simulink model "harmonic_analysis"  (R2016a)
settings: Solver=VariableStepAuto  StartTime=0.0  StopTime=Tfinal  RelTol=1e-3
values from neighbouring files (symbols this model uses):
  Ts = 0.1e-6    (= 1e-07)    [cizdir.m]
libraries: powerlib_meascontrol x80, powerlib x1
settings Model: SimulationMode=accelerator  Creator=mesutto  LastModifiedBy=mesutto

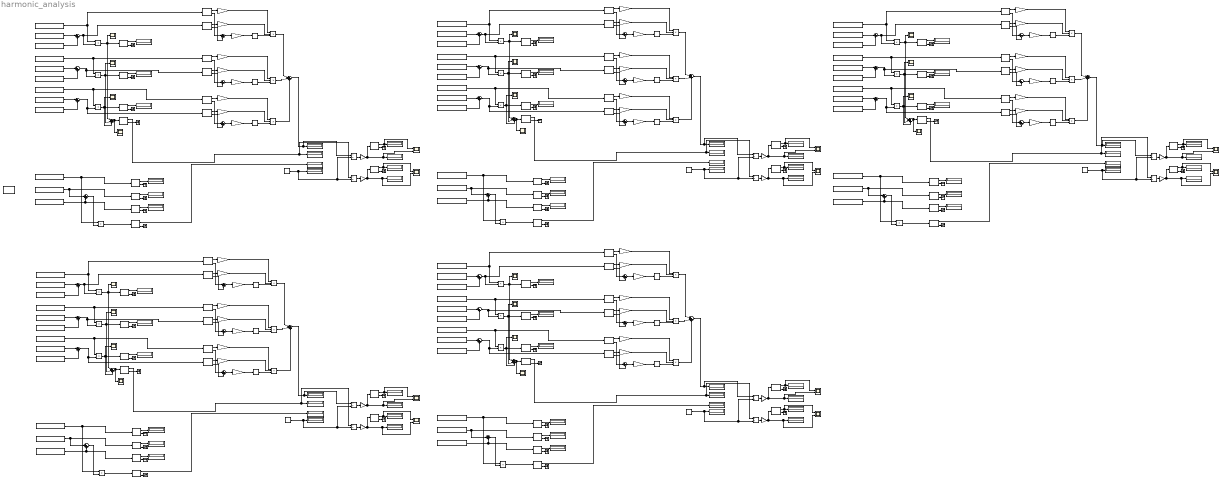
== system harmonic_analysis ==
  Constant : Constant  Value=398
  Constant1 : Constant  Value=775
  Constant2 : Constant  Value=1150
  Constant3 : Constant  Value=1530
  Constant4 : Constant  Value=1910
  Display{1..64,66..71} (70 alike) : Display
  Divide{1..4,8..9,12..13,17,19} (10 alike) : Product  Inputs=*/
  Fourier{1..6,8..12,24..29,31,36..41,43,45,50..55,57,59,64..69,71..80} (50 alike) : powerlib_meascontrol/Measurements/Fourier  Freq=freq_fourier  n=0  InInit=[0, 0]  Ts=0
  Fourier{7,13..23,30,32..35,42,44,46..49,56,58,60..63,70} (30 alike) : powerlib_meascontrol/Measurements/Fourier  Freq=50  n=1  InInit=[0, 0]  Ts=0
  From Workspace1 : FromWorkspace  VariableName=[time_DCload5*1e-3 Va_load1]  OutDataTypeStr=double  SampleTime=Ts
  From Workspace10 : FromWorkspace  VariableName=[time_DC_a1_load5*1e-3 Idc_a1_load1]  OutDataTypeStr=double  SampleTime=Ts
  From Workspace11 : FromWorkspace  VariableName=[time_DC_a2_load5*1e-3 Idc_a2_load1]  OutDataTypeStr=double  SampleTime=Ts
  From Workspace12 : FromWorkspace  VariableName=[time_DCload5*1e-3 Va_load2]  OutDataTypeStr=double  SampleTime=Ts
  From Workspace13 : FromWorkspace  VariableName=[time_DCload5*1e-3 Ic_a2_load1]  OutDataTypeStr=double  SampleTime=Ts
  From Workspace14 : FromWorkspace  VariableName=[time_DC_a1_load5*1e-3 Idc_a1_load2]  OutDataTypeStr=double  SampleTime=Ts
  From Workspace15 : FromWorkspace  VariableName=[time_DC_a2_load5*1e-3 Idc_a2_load2]  OutDataTypeStr=double  SampleTime=Ts
  From Workspace16 : FromWorkspace  VariableName=[time_DCload5*1e-3 Ic_a2_load2]  OutDataTypeStr=double  SampleTime=Ts
  From Workspace17 : FromWorkspace  VariableName=[time_DCload5*1e-3 Ia_a1_load2]  OutDataTypeStr=double  SampleTime=Ts
  From Workspace18 : FromWorkspace  VariableName=[time_DCload5*1e-3 Ia_a2_load2]  OutDataTypeStr=double  SampleTime=Ts
  From Workspace19 : FromWorkspace  VariableName=[time_DCload5*1e-3 Vb_load2]  OutDataTypeStr=double  SampleTime=Ts
  From Workspace2 : FromWorkspace  VariableName=[time_DCload5*1e-3 Ia_a1_load1]  OutDataTypeStr=double  SampleTime=Ts
  From Workspace20 : FromWorkspace  VariableName=[time_DCload5*1e-3 Ib_a1_load2]  OutDataTypeStr=double  SampleTime=Ts
  From Workspace21 : FromWorkspace  VariableName=[time_DCload5*1e-3 Ib_a2_load2]  OutDataTypeStr=double  SampleTime=Ts
  From Workspace22 : FromWorkspace  VariableName=[time_DCload5*1e-3 Vc_load2]  OutDataTypeStr=double  SampleTime=Ts
  From Workspace23 : FromWorkspace  VariableName=[time_DCload5*1e-3 Ic_a1_load2]  OutDataTypeStr=double  SampleTime=Ts
  From Workspace24 : FromWorkspace  VariableName=[time_DCload5*1e-3 Vdc_load2]  OutDataTypeStr=double  SampleTime=Ts
  From Workspace25 : FromWorkspace  VariableName=[time_DCload5*1e-3 Va_load3]  OutDataTypeStr=double  SampleTime=Ts
  From Workspace26 : FromWorkspace  VariableName=[time_DC_a1_load5*1e-3 Idc_a1_load3]  OutDataTypeStr=double  SampleTime=Ts
  From Workspace27 : FromWorkspace  VariableName=[time_DC_a2_load5*1e-3 Idc_a2_load3]  OutDataTypeStr=double  SampleTime=Ts
  From Workspace28 : FromWorkspace  VariableName=[time_DCload5*1e-3 Ic_a2_load3]  OutDataTypeStr=double  SampleTime=Ts
  From Workspace29 : FromWorkspace  VariableName=[time_DCload5*1e-3 Ia_a1_load3]  OutDataTypeStr=double  SampleTime=Ts
  From Workspace3 : FromWorkspace  VariableName=[time_DCload5*1e-3 Ia_a2_load1]  OutDataTypeStr=double  SampleTime=Ts
  From Workspace30 : FromWorkspace  VariableName=[time_DCload5*1e-3 Ia_a2_load3]  OutDataTypeStr=double  SampleTime=Ts
  From Workspace31 : FromWorkspace  VariableName=[time_DCload5*1e-3 Vb_load3]  OutDataTypeStr=double  SampleTime=Ts
  From Workspace32 : FromWorkspace  VariableName=[time_DCload5*1e-3 Ib_a1_load3]  OutDataTypeStr=double  SampleTime=Ts
  From Workspace33 : FromWorkspace  VariableName=[time_DCload5*1e-3 Ib_a2_load3]  OutDataTypeStr=double  SampleTime=Ts
  From Workspace34 : FromWorkspace  VariableName=[time_DCload5*1e-3 Vc_load3]  OutDataTypeStr=double  SampleTime=Ts
  From Workspace35 : FromWorkspace  VariableName=[time_DCload5*1e-3 Ic_a1_load3]  OutDataTypeStr=double  SampleTime=Ts
  From Workspace36 : FromWorkspace  VariableName=[time_DCload5*1e-3 Vdc_load3]  OutDataTypeStr=double  SampleTime=Ts
  From Workspace37 : FromWorkspace  VariableName=[time_DCload5*1e-3 Va_load4]  OutDataTypeStr=double  SampleTime=Ts
  From Workspace38 : FromWorkspace  VariableName=[time_DC_a1_load5*1e-3 Idc_a1_load4]  OutDataTypeStr=double  SampleTime=Ts
  From Workspace39 : FromWorkspace  VariableName=[time_DC_a2_load5*1e-3 Idc_a2_load4]  OutDataTypeStr=double  SampleTime=Ts
  From Workspace4 : FromWorkspace  VariableName=[time_DCload5*1e-3 Vb_load1]  OutDataTypeStr=double  SampleTime=Ts
  From Workspace40 : FromWorkspace  VariableName=[time_DCload5*1e-3 Ic_a2_load4]  OutDataTypeStr=double  SampleTime=Ts
  From Workspace41 : FromWorkspace  VariableName=[time_DCload5*1e-3 Ia_a1_load4]  OutDataTypeStr=double  SampleTime=Ts
  From Workspace42 : FromWorkspace  VariableName=[time_DCload5*1e-3 Ia_a2_load4]  OutDataTypeStr=double  SampleTime=Ts
  From Workspace43 : FromWorkspace  VariableName=[time_DCload5*1e-3 Vb_load4]  OutDataTypeStr=double  SampleTime=Ts
  From Workspace44 : FromWorkspace  VariableName=[time_DCload5*1e-3 Ib_a1_load4]  OutDataTypeStr=double  SampleTime=Ts
  From Workspace45 : FromWorkspace  VariableName=[time_DCload5*1e-3 Ib_a2_load4]  OutDataTypeStr=double  SampleTime=Ts
  From Workspace46 : FromWorkspace  VariableName=[time_DCload5*1e-3 Vc_load4]  OutDataTypeStr=double  SampleTime=Ts
  From Workspace47 : FromWorkspace  VariableName=[time_DCload5*1e-3 Ic_a1_load4]  OutDataTypeStr=double  SampleTime=Ts
  From Workspace48 : FromWorkspace  VariableName=[time_DCload5*1e-3 Vdc_load4]  OutDataTypeStr=double  SampleTime=Ts
  From Workspace49 : FromWorkspace  VariableName=[time_DCload5*1e-3 Va_load5]  OutDataTypeStr=double  SampleTime=Ts
  From Workspace5 : FromWorkspace  VariableName=[time_DCload5*1e-3 Ib_a1_load1]  OutDataTypeStr=double  SampleTime=Ts
  From Workspace50 : FromWorkspace  VariableName=[time_DC_a1_load5*1e-3 Idc_a1_load5]  OutDataTypeStr=double  SampleTime=Ts
  From Workspace51 : FromWorkspace  VariableName=[time_DC_a2_load5*1e-3 Idc_a2_load5]  OutDataTypeStr=double  SampleTime=Ts
  From Workspace52 : FromWorkspace  VariableName=[time_DCload5*1e-3 Ic_a2_load5]  OutDataTypeStr=double  SampleTime=Ts
  From Workspace53 : FromWorkspace  VariableName=[time_DCload5*1e-3 Ia_a1_load5]  OutDataTypeStr=double  SampleTime=Ts
  From Workspace54 : FromWorkspace  VariableName=[time_DCload5*1e-3 Ia_a2_load5]  OutDataTypeStr=double  SampleTime=Ts
  From Workspace55 : FromWorkspace  VariableName=[time_DCload5*1e-3 Vb_load5]  OutDataTypeStr=double  SampleTime=Ts
  From Workspace56 : FromWorkspace  VariableName=[time_DCload5*1e-3 Ib_a1_load5]  OutDataTypeStr=double  SampleTime=Ts
  From Workspace57 : FromWorkspace  VariableName=[time_DCload5*1e-3 Ib_a2_load5]  OutDataTypeStr=double  SampleTime=Ts
  From Workspace58 : FromWorkspace  VariableName=[time_DCload5*1e-3 Vc_load5]  OutDataTypeStr=double  SampleTime=Ts
  From Workspace59 : FromWorkspace  VariableName=[time_DCload5*1e-3 Ic_a1_load5]  OutDataTypeStr=double  SampleTime=Ts
  From Workspace6 : FromWorkspace  VariableName=[time_DCload5*1e-3 Ib_a2_load1]  OutDataTypeStr=double  SampleTime=Ts
  From Workspace60 : FromWorkspace  VariableName=[time_DCload5*1e-3 Vdc_load5]  OutDataTypeStr=double  SampleTime=Ts
  From Workspace7 : FromWorkspace  VariableName=[time_DCload5*1e-3 Vc_load1]  OutDataTypeStr=double  SampleTime=Ts
  From Workspace8 : FromWorkspace  VariableName=[time_DCload5*1e-3 Ic_a1_load1]  OutDataTypeStr=double  SampleTime=Ts
  From Workspace9 : FromWorkspace  VariableName=[time_DCload5*1e-3 Vdc_load1]  OutDataTypeStr=double  SampleTime=Ts
  Gain{1..4,32..33,45..46,58,63} (10 alike) : Gain  Gain=100
  Gain{5..6,10..11,14,19,29,38..39,42,51..52,55,64..65} (15 alike) : Gain  Gain=pi/180
  Gain{8..9,12..13,15..18,20..21,25..28,30..31,35..36,40..41,43..44,48..49,53..54,56..57,61..62} (30 alike) : Gain  Gain=1/sqrt(2)
  Product{1..5,9..11,15..17,21..24,28..31,35} (20 alike) : Product
  Product{6..8,12..14,18..20,25..27,32..34} (15 alike) : Product  Inputs=3
  Scope{1..4,9..12,17..19,24..27,32..35,40} (20 alike) : Scope
  Scope{5..8,20..21,28..29,36..37} (10 alike) : Scope  NumInputPorts=2
  Sum{1,8..10,17..19,25..26,28,34..35,37,43..44} (15 alike) : Sum  Inputs=|+-
  Sum{2,7,11,16,24,27,33,36,42,45} (10 alike) : Sum  Inputs=|+++
  Sum{3..6,12..15,20..23,29..32,38..41} (20 alike) : Sum  Inputs=|++
  Terminator{,1..49} (50 alike) : Terminator
  Trigonometric Function{1..15} (15 alike) : Trigonometry  Operator=cos
  powergui : powerlib/powergui  Priority=1  SimulationMode=Discrete  SolverType=Tustin/Backward Euler (TBE)  SampleTime=Ts  frequency=60  SPID=off  DisableSnubberDevices=off  DisableRonSwitches=off  DisableVfSwitches=off  SwTol=0  DisplayEquations=off  Interpol=off  ExternalGateDelay=off  methode=off  Ts=10  FunctionMessages=off  echomessages=off  HookPort=off  EnableUseOfTLC=off  x0status=blocks  frequencyindice=60  Pbase=100e6  ErrMax=1e-4  Iterations=50  UnitsV=kV  UnitsW=MW  buscounter=0  RestoreLinks=warning  ResistiveCurrentMeasurement=off  Frange=[0:2:500]  Ylog=off  Xlog=on  ShowGrid=off  save=off  variable=ZData  structure=Pa  ZoomFFT=off  StartTime=0.005  cycles=3  DisplayStyle=5  fundamental=100  FreqAxis=off  MaxFrequency=200000  frequencyindicesteady=1  RmsSteady=1  display=off
  wires:
  Fourier4/1 -> Display11/1
  Fourier4/2 -> Terminator/1
  From Workspace10/1 -> Sum3/1, Fourier5/1
  Fourier5/1 -> Display12/1
  Fourier5/2 -> Terminator1/1
  From Workspace11/1 -> Sum3/2, Fourier6/1
  Fourier6/1 -> Display13/1
  Fourier6/2 -> Terminator2/1
  Fourier8/2 -> Terminator4/1
  Sum3/1 -> Product2/2
  Product2/1 -> Fourier8/1
  From Workspace9/1 -> Product2/1, Fourier4/1
  From Workspace2/1 -> Sum4/1
  From Workspace3/1 -> Sum4/2
  From Workspace1/1 -> Fourier13/1, Product3/1
  From Workspace5/1 -> Sum5/1
  From Workspace6/1 -> Sum5/2
  Sum5/1 -> Product4/2, Fourier16/1
  From Workspace4/1 -> Fourier15/1, Product4/1
  From Workspace8/1 -> Sum6/1
  From Workspace13/1 -> Sum6/2
  Sum6/1 -> Fourier18/1, Product5/2
  Fourier9/1 -> Display16/1
  Fourier9/2 -> Terminator5/1
  Fourier10/1 -> Display17/1
  Fourier10/2 -> Terminator6/1
  Fourier11/1 -> Display18/1
  Fourier11/2 -> Terminator7/1
  Product3/1 -> Scope1/1, Sum7/1, Fourier9/1
  Product4/1 -> Scope2/1, Sum7/2, Fourier10/1
  Product5/1 -> Scope3/1, Sum7/3, Fourier11/1
  Fourier12/2 -> Terminator8/1
  Sum7/1 -> Scope4/1, Fourier12/1
  Fourier13/1 -> Gain8/1
  Fourier14/1 -> Gain9/1
  Sum4/1 -> Fourier14/1, Product3/2
  Fourier13/2 -> Sum8/1
  Fourier14/2 -> Sum8/2
  Sum8/1 -> Gain10/1
  Gain10/1 -> Trigonometric Function2/1
  Trigonometric Function2/1 -> Product6/3
  Gain9/1 -> Product6/2
  Gain8/1 -> Product6/1
  Fourier15/1 -> Gain12/1
  Fourier16/1 -> Gain13/1
  Fourier15/2 -> Sum9/1
  Fourier16/2 -> Sum9/2
  Sum9/1 -> Gain11/1
  Gain11/1 -> Trigonometric Function3/1
  Trigonometric Function3/1 -> Product7/3
  Gain13/1 -> Product7/2
  Gain12/1 -> Product7/1
  Fourier17/1 -> Gain15/1
  Fourier18/1 -> Gain16/1
  Fourier17/2 -> Sum10/1
  Fourier18/2 -> Sum10/2
  Sum10/1 -> Gain14/1
  Gain14/1 -> Trigonometric Function4/1
  Trigonometric Function4/1 -> Product8/3
  Gain16/1 -> Product8/2
  Gain15/1 -> Product8/1
  From Workspace7/1 -> Fourier17/1, Product5/1
  Product6/1 -> Sum11/1
  Product7/1 -> Sum11/2
  Product8/1 -> Sum11/3
  Fourier8/1 -> Display15/1
  Fourier24/1 -> Display7/1
  Fourier24/2 -> Terminator3/1
  From Workspace14/1 -> Sum12/1, Fourier25/1
  Fourier25/1 -> Display8/1
  Fourier25/2 -> Terminator9/1
  From Workspace15/1 -> Sum12/2, Fourier26/1
  Fourier26/1 -> Display9/1
  Fourier26/2 -> Terminator10/1
  Fourier27/2 -> Terminator11/1
  Sum12/1 -> Product1/2
  Product1/1 -> Fourier27/1
  From Workspace24/1 -> Product1/1, Fourier24/1
  From Workspace17/1 -> Sum13/1
  From Workspace18/1 -> Sum13/2
  From Workspace12/1 -> Fourier7/1, Product9/1
  From Workspace20/1 -> Sum14/1
  From Workspace21/1 -> Sum14/2
  Sum14/1 -> Product10/2, Fourier21/1
  From Workspace19/1 -> Fourier20/1, Product10/1
  From Workspace23/1 -> Sum15/1
  From Workspace16/1 -> Sum15/2
  Sum15/1 -> Fourier23/1, Product11/2
  Fourier28/1 -> Display14/1
  Fourier28/2 -> Terminator12/1
  Fourier1/1 -> Display20/1
  Fourier1/2 -> Terminator13/1
  Fourier2/1 -> Display22/1
  Fourier2/2 -> Terminator14/1
  Product9/1 -> Scope9/1, Sum16/1, Fourier28/1
  Product10/1 -> Scope10/1, Sum16/2, Fourier1/1
  Product11/1 -> Scope11/1, Sum16/3, Fourier2/1
  Fourier3/2 -> Terminator15/1
  Sum16/1 -> Scope12/1, Fourier3/1
  Fourier7/1 -> Gain25/1
  Fourier19/1 -> Gain26/1
  Sum13/1 -> Fourier19/1, Product9/2
  Fourier7/2 -> Sum17/1
  Fourier19/2 -> Sum17/2
  Sum17/1 -> Gain5/1
  Gain5/1 -> Trigonometric Function1/1
  Trigonometric Function1/1 -> Product12/3
  Gain26/1 -> Product12/2
  Gain25/1 -> Product12/1
  Fourier20/1 -> Gain17/1
  Fourier21/1 -> Gain18/1
  Fourier20/2 -> Sum18/1
  Fourier21/2 -> Sum18/2
  Sum18/1 -> Gain6/1
  Gain6/1 -> Trigonometric Function5/1
  Trigonometric Function5/1 -> Product13/3
  Gain18/1 -> Product13/2
  Gain17/1 -> Product13/1
  Fourier22/1 -> Gain20/1
  Fourier23/1 -> Gain21/1
  Fourier22/2 -> Sum1/1
  Fourier23/2 -> Sum1/2
  Sum1/1 -> Gain19/1
  Gain19/1 -> Trigonometric Function6/1
  Trigonometric Function6/1 -> Product14/3
  Gain21/1 -> Product14/2
  Gain20/1 -> Product14/1
  From Workspace22/1 -> Fourier22/1, Product11/1
  Product12/1 -> Sum2/1
  Product13/1 -> Sum2/2
  Product14/1 -> Sum2/3
  Fourier27/1 -> Display10/1
  Fourier36/1 -> Display40/1
  Fourier36/2 -> Terminator22/1
  From Workspace26/1 -> Sum20/1, Fourier37/1
  Fourier37/1 -> Display41/1
  Fourier37/2 -> Terminator23/1
  From Workspace27/1 -> Sum20/2, Fourier38/1
  Fourier38/1 -> Display42/1
  Fourier38/2 -> Terminator16/1
  Fourier39/2 -> Terminator17/1
  Sum20/1 -> Product15/2
  Product15/1 -> Fourier39/1
  From Workspace36/1 -> Product15/1, Fourier36/1
  From Workspace29/1 -> Sum21/1
  From Workspace30/1 -> Sum21/2
  From Workspace25/1 -> Fourier42/1, Product21/1
  From Workspace32/1 -> Sum22/1
  From Workspace33/1 -> Sum22/2
  Sum22/1 -> Product16/2, Fourier33/1
  From Workspace31/1 -> Fourier32/1, Product16/1
  From Workspace35/1 -> Sum23/1
  From Workspace28/1 -> Sum23/2
  Sum23/1 -> Fourier35/1, Product17/2
  Fourier40/1 -> Display30/1
  Fourier40/2 -> Terminator18/1
  Fourier29/1 -> Display31/1
  Fourier29/2 -> Terminator19/1
  Fourier31/1 -> Display32/1
  Fourier31/2 -> Terminator20/1
  Product21/1 -> Scope24/1, Sum24/1, Fourier40/1
  Product16/1 -> Scope17/1, Sum24/2, Fourier29/1
  Product17/1 -> Scope18/1, Sum24/3, Fourier31/1
  Fourier41/2 -> Terminator21/1
  Sum24/1 -> Scope19/1, Fourier41/1
  Fourier42/1 -> Gain35/1
  Fourier30/1 -> Gain36/1
  Sum21/1 -> Fourier30/1, Product21/2
  Fourier42/2 -> Sum25/1
  Fourier30/2 -> Sum25/2
  Sum25/1 -> Gain38/1
  Gain38/1 -> Trigonometric Function7/1
  Trigonometric Function7/1 -> Product18/3
  Gain36/1 -> Product18/2
  Gain35/1 -> Product18/1
  Fourier32/1 -> Gain27/1
  Fourier33/1 -> Gain28/1
  Fourier32/2 -> Sum26/1
  Fourier33/2 -> Sum26/2
  Sum26/1 -> Gain39/1
  Gain39/1 -> Trigonometric Function8/1
  Trigonometric Function8/1 -> Product19/3
  Gain28/1 -> Product19/2
  Gain27/1 -> Product19/1
  Fourier34/1 -> Gain30/1
  Fourier35/1 -> Gain31/1
  Fourier34/2 -> Sum19/1
  Fourier35/2 -> Sum19/2
  Sum19/1 -> Gain29/1
  Gain29/1 -> Trigonometric Function9/1
  Trigonometric Function9/1 -> Product20/3
  Gain31/1 -> Product20/2
  Gain30/1 -> Product20/1
  From Workspace34/1 -> Fourier34/1, Product17/1
  Product18/1 -> Sum27/1
  Product19/1 -> Sum27/2
  Product20/1 -> Sum27/3
  Fourier39/1 -> Display29/1
  Fourier50/1 -> Display54/1
  Fourier50/2 -> Terminator30/1
  From Workspace38/1 -> Sum29/1, Fourier51/1
  Fourier51/1 -> Display55/1
  Fourier51/2 -> Terminator31/1
  From Workspace39/1 -> Sum29/2, Fourier52/1
  Fourier52/1 -> Display56/1
  Fourier52/2 -> Terminator24/1
  Fourier53/2 -> Terminator25/1
  Sum29/1 -> Product22/2
  Product22/1 -> Fourier53/1
  From Workspace48/1 -> Product22/1, Fourier50/1
  From Workspace41/1 -> Sum30/1
  From Workspace42/1 -> Sum30/2
  From Workspace37/1 -> Fourier56/1, Product28/1
  From Workspace44/1 -> Sum31/1
  From Workspace45/1 -> Sum31/2
  Sum31/1 -> Product23/2, Fourier47/1
  From Workspace43/1 -> Fourier46/1, Product23/1
  From Workspace47/1 -> Sum32/1
  From Workspace40/1 -> Sum32/2
  Sum32/1 -> Fourier49/1, Product24/2
  Fourier54/1 -> Display44/1
  Fourier54/2 -> Terminator26/1
  Fourier43/1 -> Display45/1
  Fourier43/2 -> Terminator27/1
  Fourier45/1 -> Display46/1
  Fourier45/2 -> Terminator28/1
  Product28/1 -> Scope32/1, Sum33/1, Fourier54/1
  Product23/1 -> Scope25/1, Sum33/2, Fourier43/1
  Product24/1 -> Scope26/1, Sum33/3, Fourier45/1
  Fourier55/2 -> Terminator29/1
  Sum33/1 -> Scope27/1, Fourier55/1
  Fourier56/1 -> Gain48/1
  Fourier44/1 -> Gain49/1
  Sum30/1 -> Fourier44/1, Product28/2
  Fourier56/2 -> Sum34/1
  Fourier44/2 -> Sum34/2
  Sum34/1 -> Gain51/1
  Gain51/1 -> Trigonometric Function10/1
  Trigonometric Function10/1 -> Product25/3
  Gain49/1 -> Product25/2
  Gain48/1 -> Product25/1
  Fourier46/1 -> Gain40/1
  Fourier47/1 -> Gain41/1
  Fourier46/2 -> Sum35/1
  Fourier47/2 -> Sum35/2
  Sum35/1 -> Gain52/1
  Gain52/1 -> Trigonometric Function11/1
  Trigonometric Function11/1 -> Product26/3
  Gain41/1 -> Product26/2
  Gain40/1 -> Product26/1
  Fourier48/1 -> Gain43/1
  Fourier49/1 -> Gain44/1
  Fourier48/2 -> Sum28/1
  Fourier49/2 -> Sum28/2
  Sum28/1 -> Gain42/1
  Gain42/1 -> Trigonometric Function12/1
  Trigonometric Function12/1 -> Product27/3
  Gain44/1 -> Product27/2
  Gain43/1 -> Product27/1
  From Workspace46/1 -> Fourier48/1, Product24/1
  Product25/1 -> Sum36/1
  Product26/1 -> Sum36/2
  Product27/1 -> Sum36/3
  Fourier53/1 -> Display43/1
  Fourier64/1 -> Display68/1
  Fourier64/2 -> Terminator38/1
  From Workspace50/1 -> Sum38/1, Fourier65/1
  Fourier65/1 -> Display69/1
  Fourier65/2 -> Terminator39/1
  From Workspace51/1 -> Sum38/2, Fourier66/1
  Fourier66/1 -> Display70/1
  Fourier66/2 -> Terminator32/1
  Fourier67/2 -> Terminator33/1
  Sum38/1 -> Product29/2
  Product29/1 -> Fourier67/1
  From Workspace60/1 -> Product29/1, Fourier64/1
  From Workspace53/1 -> Sum39/1
  From Workspace54/1 -> Sum39/2
  From Workspace49/1 -> Fourier70/1, Product35/1
  From Workspace56/1 -> Sum40/1
  From Workspace57/1 -> Sum40/2
  Sum40/1 -> Product30/2, Fourier61/1
  From Workspace55/1 -> Fourier60/1, Product30/1
  From Workspace59/1 -> Sum41/1
  From Workspace52/1 -> Sum41/2
  Sum41/1 -> Fourier63/1, Product31/2
  Fourier68/1 -> Display58/1
  Fourier68/2 -> Terminator34/1
  Fourier57/1 -> Display59/1
  Fourier57/2 -> Terminator35/1
  Fourier59/1 -> Display60/1
  Fourier59/2 -> Terminator36/1
  Product35/1 -> Scope40/1, Sum42/1, Fourier68/1
  Product30/1 -> Scope33/1, Sum42/2, Fourier57/1
  Product31/1 -> Scope34/1, Sum42/3, Fourier59/1
  Fourier69/1 -> Divide17/1, Display61/1
  Fourier69/2 -> Terminator37/1
  Sum42/1 -> Scope35/1, Fourier69/1
  Fourier70/1 -> Gain61/1
  Fourier58/1 -> Gain62/1
  Sum39/1 -> Fourier58/1, Product35/2
  Fourier70/2 -> Sum43/1
  Fourier58/2 -> Sum43/2
  Sum43/1 -> Gain64/1
  Gain64/1 -> Trigonometric Function13/1
  Trigonometric Function13/1 -> Product32/3
  Gain62/1 -> Product32/2
  Gain61/1 -> Product32/1
  Fourier60/1 -> Gain53/1
  Fourier61/1 -> Gain54/1
  Fourier60/2 -> Sum44/1
  Fourier61/2 -> Sum44/2
  Sum44/1 -> Gain65/1
  Gain65/1 -> Trigonometric Function14/1
  Trigonometric Function14/1 -> Product33/3
  Gain54/1 -> Product33/2
  Gain53/1 -> Product33/1
  Fourier62/1 -> Gain56/1
  Fourier63/1 -> Gain57/1
  Fourier62/2 -> Sum37/1
  Fourier63/2 -> Sum37/2
  Sum37/1 -> Gain55/1
  Gain55/1 -> Trigonometric Function15/1
  Trigonometric Function15/1 -> Product34/3
  Gain57/1 -> Product34/2
  Gain56/1 -> Product34/1
  From Workspace58/1 -> Fourier62/1, Product31/1
  Product32/1 -> Sum45/1
  Product33/1 -> Sum45/2
  Product34/1 -> Sum45/3
  Sum45/1 -> Divide19/1, Display63/1
  Fourier67/1 -> Display57/1
  Constant4/1 -> Divide17/2, Divide19/2, Display67/1
  Gain63/1 -> Fourier71/1, Scope36/2, Display64/1
  Divide19/1 -> Gain63/1
  Divide17/1 -> Gain58/1
  Gain58/1 -> Scope37/2, Display66/1, Fourier72/1
  Fourier71/1 -> Scope36/1, Display71/1
  Fourier71/2 -> Terminator40/1
  Fourier72/1 -> Scope37/1, Display62/1
  Fourier72/2 -> Terminator41/1
  Fourier55/1 -> Divide12/1, Display47/1
  Sum36/1 -> Divide13/1, Display49/1
  Constant3/1 -> Divide12/2, Divide13/2, Display53/1
  Gain46/1 -> Fourier73/1, Scope28/2, Display50/1
  Divide13/1 -> Gain46/1
  Divide12/1 -> Gain45/1
  Gain45/1 -> Scope29/2, Display51/1, Fourier74/1
  Fourier73/1 -> Scope28/1, Display52/1
  Fourier73/2 -> Terminator42/1
  Fourier74/1 -> Scope29/1, Display48/1
  Fourier74/2 -> Terminator43/1
  Fourier41/1 -> Divide8/1, Display33/1
  Sum27/1 -> Divide9/1, Display35/1
  Constant2/1 -> Divide8/2, Divide9/2, Display39/1
  Gain33/1 -> Fourier75/1, Scope20/2, Display36/1
  Divide9/1 -> Gain33/1
  Divide8/1 -> Gain32/1
  Gain32/1 -> Scope21/2, Display37/1, Fourier76/1
  Fourier75/1 -> Scope20/1, Display38/1
  Fourier75/2 -> Terminator44/1
  Fourier76/1 -> Scope21/1, Display34/1
  Fourier76/2 -> Terminator45/1
  Fourier12/1 -> Divide1/1, Display19/1
  Sum11/1 -> Divide2/1, Display21/1
  Constant/1 -> Divide1/2, Divide2/2, Display1/1
  Gain2/1 -> Fourier77/1, Scope5/2, Display3/1
  Divide2/1 -> Gain2/1
  Divide1/1 -> Gain1/1
  Gain1/1 -> Scope6/2, Display4/1, Fourier78/1
  Fourier77/1 -> Scope5/1, Display5/1
  Fourier77/2 -> Terminator46/1
  Fourier78/1 -> Scope6/1, Display2/1
  Fourier78/2 -> Terminator47/1
  Fourier3/1 -> Divide3/1, Display23/1
  Sum2/1 -> Divide4/1, Display25/1
  Constant1/1 -> Divide3/2, Divide4/2, Display6/1
  Gain4/1 -> Fourier79/1, Scope7/2, Display26/1
  Divide4/1 -> Gain4/1
  Divide3/1 -> Gain3/1
  Gain3/1 -> Scope8/2, Display27/1, Fourier80/1
  Fourier79/1 -> Scope7/1, Display28/1
  Fourier79/2 -> Terminator48/1
  Fourier80/1 -> Scope8/1, Display24/1
  Fourier80/2 -> Terminator49/1
